simulink model "v2_new_5d_openloop"  (Simulink 7.8)
settings: Solver=ode15s  StartTime=0.0  StopTime=21600  MaxStep=1  MinStep=1e-12  RelTol=1e-10
settings Model: Creator=jahansha  LastModifiedBy=matslie
settings DebuggingCC: FcnCallInpInsideContextMsg=Use local settings

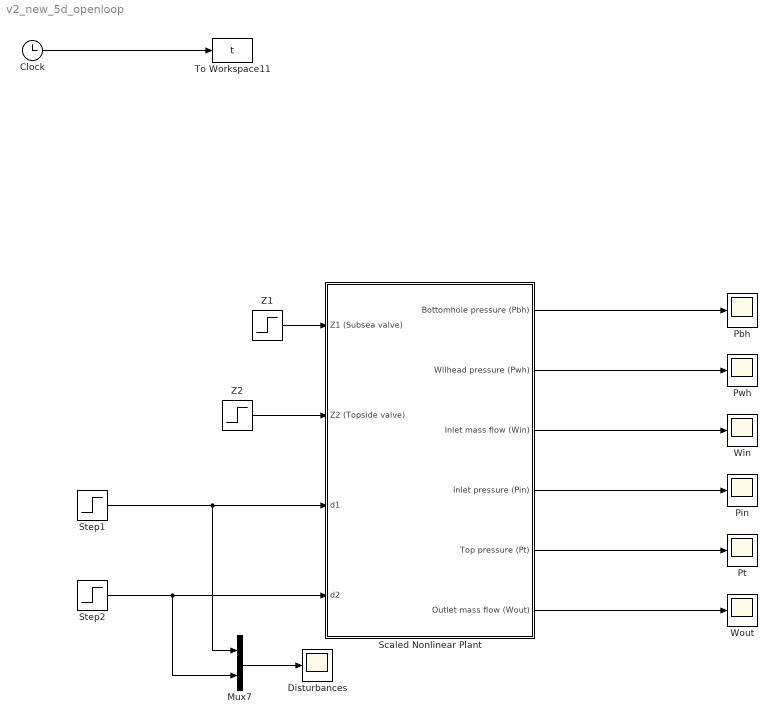
== system v2_new_5d_openloop ==
  Clock : Clock
  Disturbances : Scope
      settings: TimeRange=8000  YMin=1.38778e-017  YMax=0.275  SaveName=ScopeData5
  Mux7 : Mux  Inputs=2
  Pbh : Scope
      settings: TimeRange=100000  YMin=-0.1915  YMax=-0.184  SaveName=ScopeData3
  Pin : Scope
      settings: TimeRange=8000  YMin=0.105  YMax=0.113  SaveName=ScopeData7
  Pt : Scope
      settings: TimeRange=8000  YMin=0.105  YMax=0.113
  Pwh : Scope
      settings: TimeRange=10000  YMin=-0.0275  YMax=-0.0075  SaveName=ScopeData4
  Scaled Nonlinear Plant : Subsystem
  Step1 : Step  Time=10000  After=0  SampleTime=0
  Step2 : Step  Time=20000  After=0  SampleTime=0
  To Workspace11 : ToWorkspace  VariableName=t  SampleTime=-1  SaveFormat=Array
  Win : Scope
      settings: YMin=0.225  YMax=0.55  SaveName=ScopeData2
  Wout : Scope
      settings: TimeRange=100000  YMin=-0.6  YMax=1.4  SaveName=ScopeData6
  Z1 : Step  Time=7200  Before=0.1  After=0.1  SampleTime=0
  Z2 : Step  Time=7200  Before=0.035  After=0.04  SampleTime=0
  wires:
  Mux7/1 -> Disturbances/1
  Step1/1 -> Mux7/1, Scaled Nonlinear Plant/3(d1)
  Step2/1 -> Mux7/2, Scaled Nonlinear Plant/4(d2)
  Scaled Nonlinear Plant/1(Bottomhole pressure (Pbh)) -> Pbh/1
  Scaled Nonlinear Plant/2(Wllhead pressure (Pwh)) -> Pwh/1
  Scaled Nonlinear Plant/3(Inlet mass flow (Win)) -> Win/1
  Scaled Nonlinear Plant/4(Inlet pressure (Pin)) -> Pin/1
  Scaled Nonlinear Plant/5(Top pressure (Pt)) -> Pt/1
  Scaled Nonlinear Plant/6(Outlet mass flow (Wout)) -> Wout/1
  Z2/1 -> Scaled Nonlinear Plant/2(Z2 (Topside valve))
  Z1/1 -> Scaled Nonlinear Plant/1(Z1 (Subsea valve))
  Clock/1 -> To Workspace11/1

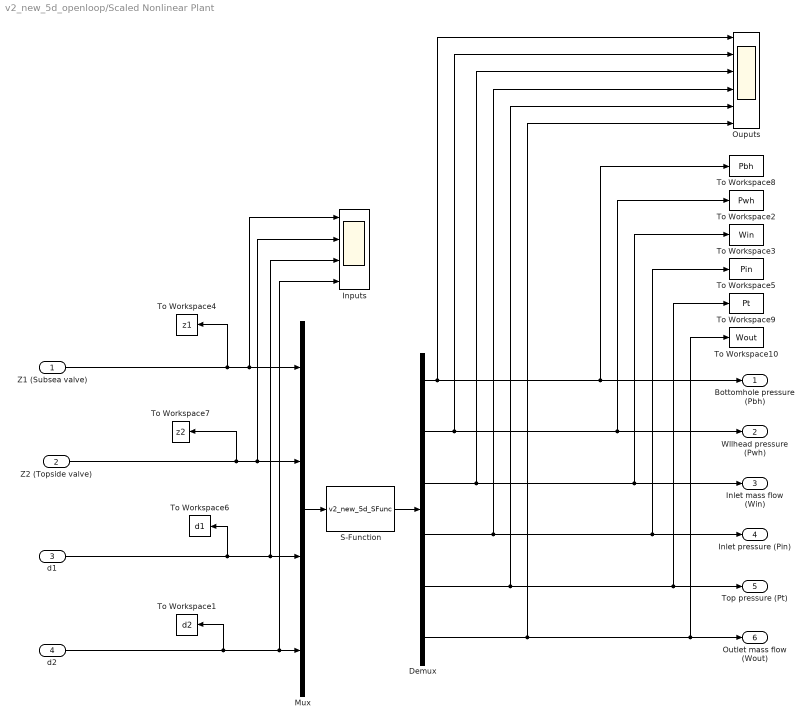
== system v2_new_5d_openloop/Scaled Nonlinear Plant ==
  Z1 (Subsea valve) : Inport
  Z2 (Topside valve) : Inport  Port=2
  d1 : Inport  Port=3
  d2 : Inport  Port=4
  Demux : Demux  Outputs=6
  Inputs : Scope  NumInputPorts=4
      settings: TimeRange=8000  YMin=-1~-5~-5~-5  YMax=1~5~5~5  SaveName=ScopeData9
  Mux : Mux
  Ouputs : Scope  NumInputPorts=6
      settings: TimeRange=100000  YMin=279.857~71.1957~11.0392~71.1306~51.6171~11.4892  YMax=279.857~71.1957~11.0392~71.1307~51.6171~11.4892  SaveName=ScopeData10
  S-Function : S-Function  FunctionName=v2_new_5d_SFunc  EnableBusSupport=off
  To Workspace1 : ToWorkspace  VariableName=d2  SampleTime=-1  SaveFormat=Array
  To Workspace10 : ToWorkspace  VariableName=Wout  SampleTime=-1  SaveFormat=Array
  To Workspace2 : ToWorkspace  VariableName=Pwh  SampleTime=-1  SaveFormat=Array
  To Workspace3 : ToWorkspace  VariableName=Win  SampleTime=-1  SaveFormat=Array
  To Workspace4 : ToWorkspace  VariableName=z1  SampleTime=-1  SaveFormat=Array
  To Workspace5 : ToWorkspace  VariableName=Pin  SampleTime=-1  SaveFormat=Array
  To Workspace6 : ToWorkspace  VariableName=d1  SampleTime=-1  SaveFormat=Array
  To Workspace7 : ToWorkspace  VariableName=z2  SampleTime=-1  SaveFormat=Array
  To Workspace8 : ToWorkspace  VariableName=Pbh  SampleTime=-1  SaveFormat=Array
  To Workspace9 : ToWorkspace  VariableName=Pt  SampleTime=-1  SaveFormat=Array
  Bottomhole pressure (Pbh) : Outport
  Wllhead pressure (Pwh) : Outport  Port=2
  Inlet mass flow (Win) : Outport  Port=3
  Inlet pressure (Pin) : Outport  Port=4
  Top pressure (Pt) : Outport  Port=5
  Outlet mass flow (Wout) : Outport  Port=6
  wires:
  Mux/1 -> S-Function/1
  S-Function/1 -> Demux/1
  Demux/1 -> Ouputs/1, Bottomhole pressure (Pbh)/1, To Workspace8/1
  Demux/2 -> Ouputs/2, Wllhead pressure (Pwh)/1, To Workspace2/1
  Demux/3 -> Ouputs/3, Inlet mass flow (Win)/1, To Workspace3/1
  Demux/4 -> Ouputs/4, Inlet pressure (Pin)/1, To Workspace5/1
  Z1 (Subsea valve)/1 -> Mux/1, To Workspace4/1, Inputs/1
  d1/1 -> To Workspace6/1, Mux/3, Inputs/3
  d2/1 -> To Workspace1/1, Mux/4, Inputs/4
  Z2 (Topside valve)/1 -> To Workspace7/1, Mux/2, Inputs/2
  Demux/5 -> Ouputs/5, Top pressure (Pt)/1, To Workspace9/1
  Demux/6 -> Ouputs/6, Outlet mass flow (Wout)/1, To Workspace10/1
